simulink model "Task_1F"  (R2022a)
settings: Solver=VariableStepAuto  StartTime=0.0  StopTime=t_in(end) + 1  RelTol=1e-3
settings Model: Creator=jpcas  LastModifiedBy=jpcas

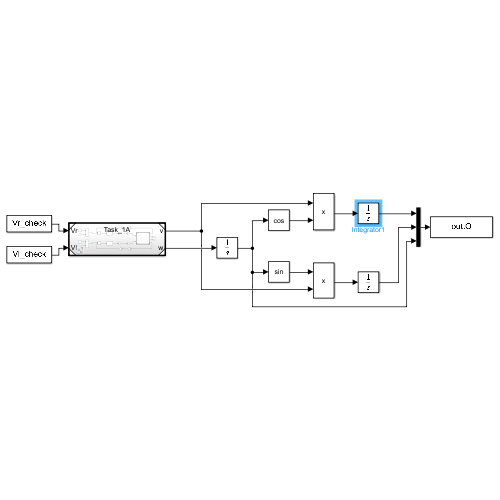
[thumbnail: Simulink's stored preview of the top-level diagram]
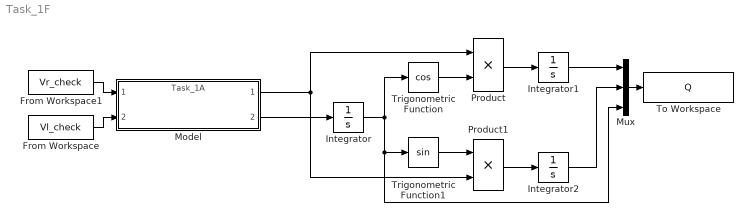
== system Task_1F ==
  From Workspace : FromWorkspace  VariableName=Vl_check
  From Workspace1 : FromWorkspace  VariableName=Vr_check
  Integrator : Integrator  InitialCondition=pi
  Integrator1 : Integrator
  Integrator2 : Integrator
  Model : ModelReference  ModelNameDialog=Task_1A  SimulationMode=Normal  ModelReferenceVersion=1.12
  Mux : Mux  Inputs=3
  Product : Product
  Product1 : Product
  To Workspace : ToWorkspace  VariableName=Q  SaveFormat=Timeseries  SampleTime=-1
  Trigonometric Function : Trigonometry  Operator=cos
  Trigonometric Function1 : Trigonometry
  wires:
  From Workspace/1 -> Model/2
  From Workspace1/1 -> Model/1
  Mux/1 -> To Workspace/1
  Model/1 -> Product1/2, Product/1
  Model/2 -> Integrator/1
  Integrator/1 -> Mux/3, Trigonometric Function1/1, Trigonometric Function/1
  Trigonometric Function/1 -> Product/2
  Trigonometric Function1/1 -> Product1/1
  Product1/1 -> Integrator2/1
  Product/1 -> Integrator1/1
  Integrator1/1 -> Mux/1
  Integrator2/1 -> Mux/2
